simulink library "FadingComponent"  (Simulink 7.4)
settings: Solver=ode45  StartTime=0.0  StopTime=10.0  RelTol=1e-3
libraries: simulink x2
settings Model: Creator=anvo  LastModifiedBy=anvo

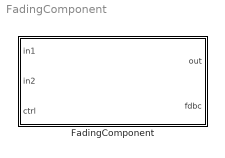
== system FadingComponent ==
  FadingComponent : Subsystem  Tag=id=_usUaEFm8EeOAF8aRyJT_5g

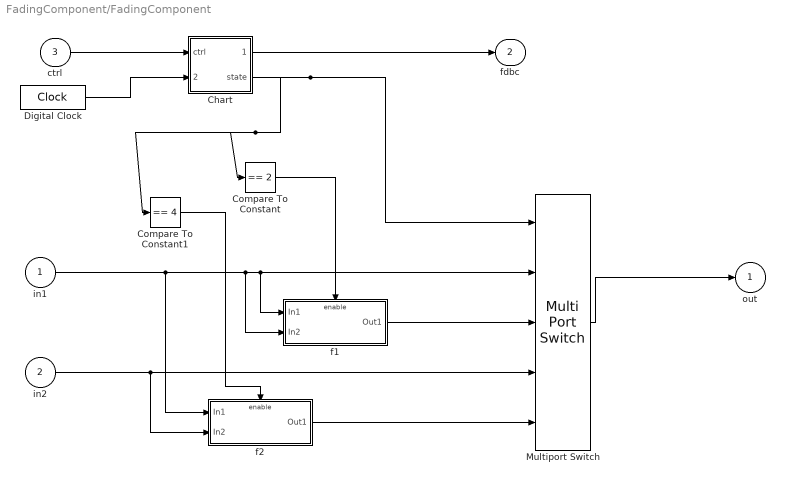
== system FadingComponent/FadingComponent ==
  in1 : Inport  Tag=id=_Hp_8cFm5EeOAF8aRyJT_5g  OutDataType=fixdt(1, 16)  OutScaling=2^0
  in2 : Inport  Tag=id=_HqH4QFm5EeOAF8aRyJT_5g  Port=2  OutDataType=fixdt(1, 16)  OutScaling=2^0
  ctrl : Inport  Tag=id=_lAWZNlm-EeOAF8aRyJT_5g  Port=3  OutDataType=fixdt(1, 16)  OutScaling=2^0
  Chart : Stateflow chart
  Compare To Constant : simulink/Logic and Bit Operations/Compare To Constant  SystemSampleTime=-1  relop===  const=2  LogicOutDataTypeMode=uint8
  Compare To Constant1 : simulink/Logic and Bit Operations/Compare To Constant  SystemSampleTime=-1  relop===  const=4  LogicOutDataTypeMode=uint8
  Digital Clock : DigitalClock  SampleTime=0.001
  Multiport Switch : MultiPortSwitch  Inputs=4  OutDataType=fixdt(1, 16)  OutScaling=2^0
  f1 : Subsystem  TreatAsAtomicUnit=on
  f2 : Subsystem  TreatAsAtomicUnit=on
  out : Outport  Tag=id=_HqWhwFm5EeOAF8aRyJT_5g  OutDataType=fixdt(1, 16)  OutScaling=2^0
  fdbc : Outport  Tag=id=_lAWZOFm-EeOAF8aRyJT_5g  Port=2  OutDataType=fixdt(1, 16)  OutScaling=2^0
  wires:
  ctrl/1 -> Chart/1(ctrl)
  Chart/1(status) -> fdbc/1
  Multiport Switch/1 -> out/1
  in1/1 -> f2/1(In1), Multiport Switch/2, f1/1(In1), f1/2(In2)
  in2/1 -> Multiport Switch/4, f2/2(In2)
  Chart/2(state) -> Multiport Switch/1, Compare To Constant/1, Compare To Constant1/1
  f1/1(Out1) -> Multiport Switch/3
  f2/1(Out1) -> Multiport Switch/5
  Compare To Constant/1 -> f1/Enable
  Compare To Constant1/1 -> f2/Enable
  Digital Clock/1 -> Chart/2(clockSignal)

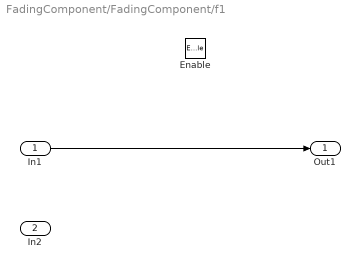
== system FadingComponent/FadingComponent/f1 ==
  In1 : Inport  OutDataType=fixdt(1, 16)  OutScaling=2^0
  In2 : Inport  Port=2  OutDataType=fixdt(1, 16)  OutScaling=2^0
  Enable : EnablePort
  Out1 : Outport  OutDataType=fixdt(1, 16)  OutScaling=2^0
  wires:
  In1/1 -> Out1/1

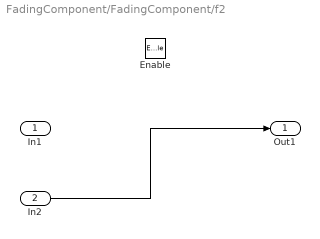
== system FadingComponent/FadingComponent/f2 ==
  In1 : Inport  OutDataType=fixdt(1, 16)  OutScaling=2^0
  In2 : Inport  Port=2  OutDataType=fixdt(1, 16)  OutScaling=2^0
  Enable : EnablePort
  Out1 : Outport  OutDataType=fixdt(1, 16)  OutScaling=2^0
  wires:
  In2/1 -> Out1/1

== stateflow chart FadingComponent/Chart ==
  state Static1
    entry: status=0;
    state=1;
  state Fading1
    entry: status=1;
    c=reset();
    state=2;
  state Fading2
    entry: status=1;
    c=reset();
    state=4;
  state Static2
    entry: status=0;
    state=3;
  (default) -> Static1
  Static1 -> Fading1 : [ctrl==1]
  Fading1 -> Static2 : [time(c) > 250]
  Static2 -> Fading2 : [ctrl==1]
  Fading2 -> Static1 : [time(c) > 250]
  data: clock function_output double; clock function_input double; logicalTime function_output uint32; ctrl input double; status output double; state output double; clockSignal input double; c local double
  function clock = reset():
    | function clock = reset() 
    | 
    |  %set clock variable to current time 
    | 
    |  clock = clockSignal;
  function logicalTime = time(clock):
    | function logicalTime = time(clock) 
    | 
    |  sample = 0.001;  % the sample time of the system clock 
    | 
    |  %convert to pass units of time after last reset 
    | 
    |  logicalTime = uint32((clockSignal - clock)/sample);
